simulink subsystem "Attitude_Control"  (R2024b)
settings: Solver=VariableStepAuto  StartTime=0.0  StopTime=10.0  RelTol=1e-3
libraries: aerolibutil x1, eeGeneralControl x1
settings Model: Creator=thesa  LastModifiedBy=jack
settings RTWCC: GPUComputeCapability=3.5

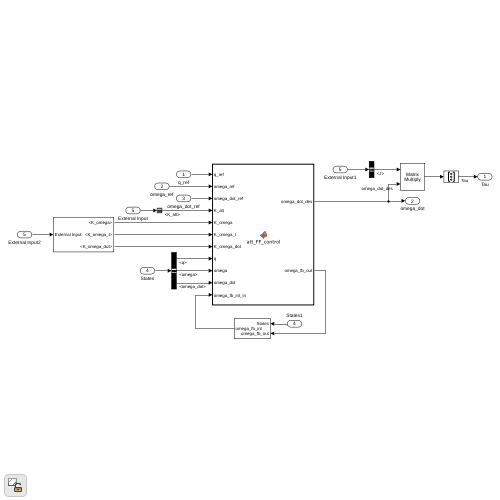
[thumbnail: Simulink's stored preview of the top-level diagram]
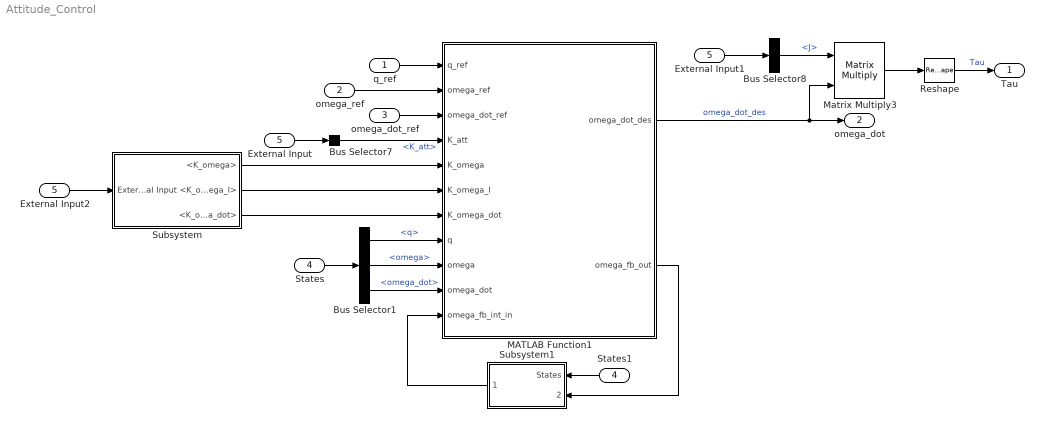
== system Attitude_Control ==
  q_ref : Inport
  omega_ref : Inport  Port=2
  omega_dot_ref : Inport  Port=3
  States : Inport  Port=4
  External Input : Inport  Port=5
  Bus Selector1 : BusSelector  OutputSignals=q,omega,omega_dot
  Bus Selector7 : BusSelector  OutputSignals=Control Gains.K_att
  Bus Selector8 : BusSelector  OutputSignals=Vehicle Parameters.J
  External Input1 : InportShadow  Port=5
  External Input2 : InportShadow  Port=5
  MATLAB Function1 : MATLAB Function  TreatAsAtomicUnit=on
  Matrix Multiply3 : Product  Multiplication=Matrix(*)
  Reshape : Reshape  OutputDimensionality=Column vector (2-D)
  States1 : InportShadow  Port=4
  Subsystem : Subsystem
  Subsystem1 : Subsystem
  Tau : Outport
  omega_dot : Outport  Port=2
  wires:
  Bus Selector1/1 -> MATLAB Function1/8(q)  "<q>"
  Bus Selector7/1 -> MATLAB Function1/4(K_att)  "<K_att>"
  Bus Selector8/1 -> Matrix Multiply3/1  "<J>"
  omega_ref/1 -> MATLAB Function1/2(omega_ref)
  Matrix Multiply3/1 -> Reshape/1
  MATLAB Function1/1(omega_dot_des) -> omega_dot/1, Matrix Multiply3/2  "omega_dot_des"
  Bus Selector1/2 -> MATLAB Function1/9(omega)  "<omega>"
  q_ref/1 -> MATLAB Function1/1(q_ref)
  Reshape/1 -> Tau/1  "Tau"
  States/1 -> Bus Selector1/1
  External Input1/1 -> Bus Selector8/1
  External Input/1 -> Bus Selector7/1
  Bus Selector1/3 -> MATLAB Function1/10(omega_dot)  "<omega_dot>"
  omega_dot_ref/1 -> MATLAB Function1/3(omega_dot_ref)
  External Input2/1 -> Subsystem/1(External Input)
  Subsystem/1(<K_omega>) -> MATLAB Function1/5(K_omega)
  Subsystem/3(<K_omega_dot>) -> MATLAB Function1/7(K_omega_dot)
  MATLAB Function1/2(omega_fb_out) -> Subsystem1/2(omega_fb_out)
  States1/1 -> Subsystem1/1(States)
  Subsystem/2(<K_omega_I>) -> MATLAB Function1/6(K_omega_I)
  Subsystem1/1(omega_fb_int) -> MATLAB Function1/11(omega_fb_int_in)

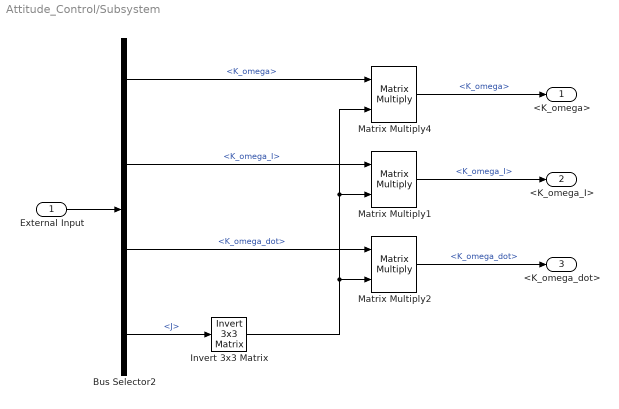
== system Attitude_Control/Subsystem ==
  External Input : Inport
  Bus Selector2 : BusSelector  OutputSignals=Control Gains.K_omega,Control Gains.K_omega_I,Control Gains.K_omega_dot,Vehicle Parameters.J
  Invert 3x3 Matrix : aerolibutil/Invert  3x3 Matrix
  Matrix Multiply1 : Product  Multiplication=Matrix(*)
  Matrix Multiply2 : Product  Multiplication=Matrix(*)
  Matrix Multiply4 : Product  Multiplication=Matrix(*)
  <K_omega> : Outport
  <K_omega_I> : Outport  Port=2
  <K_omega_dot> : Outport  Port=3
  wires:
  Matrix Multiply1/1 -> <K_omega_I>/1  "<K_omega_I>"
  Bus Selector2/2 -> Matrix Multiply1/1  "<K_omega_I>"
  Invert 3x3 Matrix/1 -> Matrix Multiply2/2, Matrix Multiply4/2, Matrix Multiply1/2
  Bus Selector2/4 -> Invert 3x3 Matrix/1  "<J>"
  Matrix Multiply2/1 -> <K_omega_dot>/1  "<K_omega_dot>"
  Bus Selector2/1 -> Matrix Multiply4/1  "<K_omega>"
  Matrix Multiply4/1 -> <K_omega>/1  "<K_omega>"
  Bus Selector2/3 -> Matrix Multiply2/1  "<K_omega_dot>"
  External Input/1 -> Bus Selector2/1

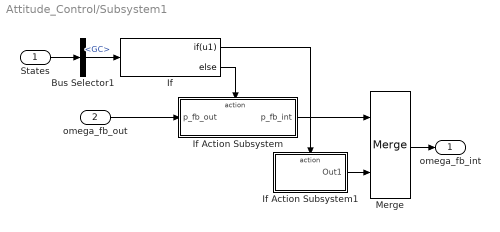
== system Attitude_Control/Subsystem1 ==
  States : Inport
  omega_fb_out : Inport  Port=2
  Bus Selector1 : BusSelector  OutputSignals=GC
  If : If  IfExpression=u1
  If Action Subsystem : Subsystem  TreatAsAtomicUnit=on
  If Action Subsystem1 : Subsystem  TreatAsAtomicUnit=on
  Merge : Merge
  omega_fb_int : Outport
  wires:
  Bus Selector1/1 -> If/1  "<GC>"
  If/1 -> If Action Subsystem1/Action
  omega_fb_out/1 -> If Action Subsystem/1(p_fb_out)
  States/1 -> Bus Selector1/1
  If/2 -> If Action Subsystem/Action
  If Action Subsystem/1(p_fb_int) -> Merge/1
  If Action Subsystem1/1(Out1) -> Merge/2
  Merge/1 -> omega_fb_int/1

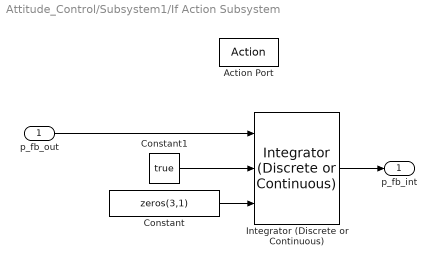
== system Attitude_Control/Subsystem1/If Action Subsystem ==
  p_fb_out : Inport
  Action Port : ActionPort  InitializeStates=reset
  Constant : Constant  Value=zeros(3,1)
  Constant1 : Constant  Value=true
  Integrator (Discrete or Continuous) : eeGeneralControl/Integrator (Discrete or Continuous)  LabelModeActiveChoice=Discrete  ExternalReset=either  LimitType=Anti-windup  B=0.5  A=-0.5  Ts=-1
      settings: LibrarySourceBlock=|
      | ee_sl_lib/General Control/Integrator
      | (Discrete or Continuous)
  p_fb_int : Outport
  wires:
  Constant1/1 -> Integrator (Discrete or Continuous)/2
  Integrator (Discrete or Continuous)/1 -> p_fb_int/1
  Constant/1 -> Integrator (Discrete or Continuous)/3
  p_fb_out/1 -> Integrator (Discrete or Continuous)/1

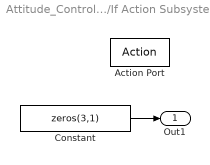
== system Attitude_Control/Subsystem1/If Action Subsystem1 ==
  Action Port : ActionPort
  Constant : Constant  Value=zeros(3,1)
  Out1 : Outport
  wires:
  Constant/1 -> Out1/1

== matlab function Attitude_Control/MATLAB Function1 ==
  data: omega_dot_des output; q_ref input; omega_ref input; omega_dot_ref input; K_att input; K_omega input; K_omega_I input; K_omega_dot input; q input; omega input; omega_dot input; omega_fb_int_in input; omega_fb_out output
function [omega_dot_des, omega_fb_out]  = att_FF_control(...
    q_ref, omega_ref, omega_dot_ref, ...
    K_att, K_omega, K_omega_I, K_omega_dot,...
    q, omega, omega_dot, omega_fb_int_in)%#codegen

%% inputs %%
K_att_ = ...
    K_att(1:3,1:3);             % attitude controller gains
K_omega_ = ...
    K_omega(1:3,1:3);           % body rate controller gains
K_omega_I_ = ...
    K_omega_I(1:3,1:3);           % body rate Integral controller gains
K_omega_dot_ = ...
    K_omega_dot(1:3,1:3);       % angular acceleration controller gains

q_ref_ = q_ref(1,1:4);          % reference attitude quaternian
omega_ref_ = ...
    omega_ref(1:3,1);           %[rad/s] reference body rates
omega_dot_ref_ = ...
    omega_dot_ref(1:3,1);       %[rad/s2] reference angular acceleration
q_ = q(1,1:4);                  %[qw qx qy qz] estimated quaternian attitude
omega_ = omega(1:3,1);          %[rad/s] estimated body rotation rates
omega_dot_ = omega_dot(1:3,1);  %[rad/s2] estimated angular acceleration
omega_fb_int_in_ = omega_fb_int_in(1:3,1);

%% outputs %%
omega_dot_des = zeros(3,1);
omega_fb_out = zeros(3,1);

%% Attitude Control %%
rate_ref = att_quat_control(q_, q_ref_, omega_ref_(3), diag(K_att_), [1000, 1000, 1000]);

% add the rate control:
omega_fb_ = (rate_ref - omega_);
omega_fb_out(:) = omega_fb_(:);

omega_dot_fb_ = (omega_dot_ref_ - omega_dot_);
omega_dot_des(:) = K_omega_ * omega_fb_(:) + K_omega_dot_*omega_dot_fb_(:) + K_omega_I_*omega_fb_int_in_;
end
